simulink model "dynamic_simulation_control_old"  (R2017b)
settings: Solver=FixedStepAuto  StartTime=0.0  StopTime=20.0  FixedStep=1e-3  RelTol=1e-3
values from neighbouring files (symbols this model uses):
  B_env = [0;10;0]    [init_dynamic_sim.m]
  dth0 = [0; 0; 0]    [dynamic_simulation.m]    (also in init_dynamic_sim.m = dq0)
  fz0 = 0    [init_dynamic_sim.m]
  K = 0.015    [init_dynamic_sim.m]
  K_env = [0;100;0]    [init_dynamic_sim.m]
  Ki = 0.08    [init_dynamic_sim.m]
  Kj = [1;1;1]*5    [init_dynamic_sim.m]
  Kjd = [1;1;1]*0.1    [init_dynamic_sim.m]
  Kv = [2500;1500;2000]/256    [init_dynamic_sim.m]
  Kvi = [3000;900;1000]/65536    [init_dynamic_sim.m]
  Kx = [20;0;0]    [init_dynamic_sim.m]
  Kxi = [0;0;0]    [init_dynamic_sim.m]
  M_env = [0;1;0]    [init_dynamic_sim.m]
  ry0 = acos(r(1,1))    [init_dynamic_sim.m]
  th0 = 0    [DGM_youBot.m]    (also in DGM_youBot_sym.m; dynamic_simulation.m = q_dh - (q0_kuka - q_rob); init_dynamic_sim.m = theta_DH(2:4) - (q0 - KUKA_offset(2:4)))
  thmax = theta_DH - (qmin - KUKA_offset)    [init_dynamic_sim.m]
  thmin = theta_DH - (qmax - KUKA_offset)    [init_dynamic_sim.m]
  x0 = p0(1)    [init_dynamic_sim.m]    (also in jacobian_computation.m = 0.033)
  z0 = 0.3    [dynamic_simulation.m]    (also in init_dynamic_sim.m = p0(3); jacobian_computation.m = 0.147)
undefined symbols (not defined in the file or in its folder): p0
libraries: aerolibutil x1
settings Model: Creator=fortineau_vin  LastModifiedBy=fortineau_vin

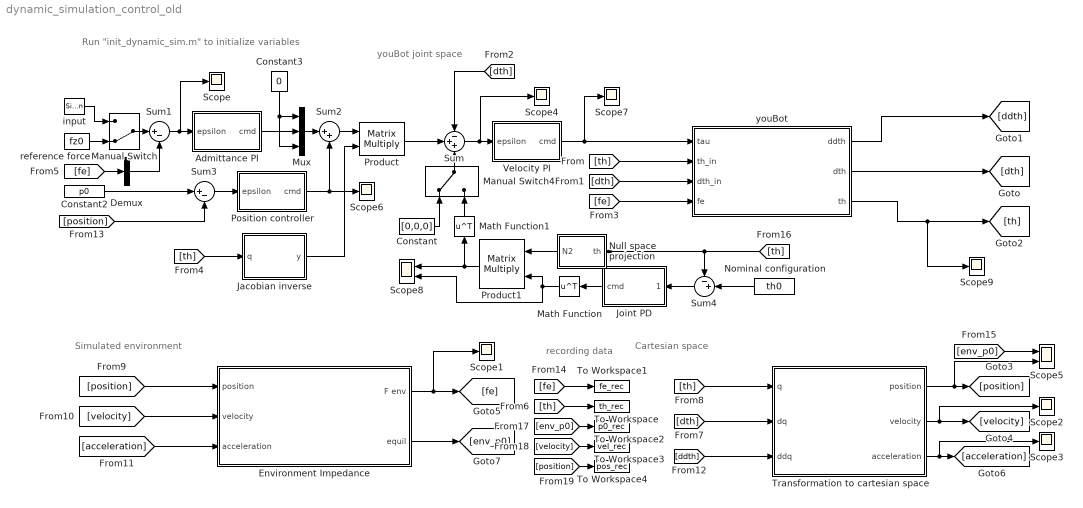
== system dynamic_simulation_control_old ==
  note: recording data
  note: Run "init_dynamic_sim.m" to initialize variables
  note: youBot joint space
  note: Simulated environment
  note: Cartesian space
  Admittance PI : Subsystem
  Constant : Constant  Value=[0,0,0]
  Constant2 : Constant  Value=p0
  Constant3 : Constant  Value=0
  Demux : Demux  Outputs=3
  "Environment Impedance " : Subsystem
  Jacobian inverse : MATLAB Function  TreatAsAtomicUnit=on
  Joint PD : Subsystem
  Manual Switch : ManualSwitch  CurrentSetting=0
  Manual Switch4 : ManualSwitch
  Math Function : Math  Operator=transpose  SaturateOnIntegerOverflow=on
  Math Function1 : Math  Operator=transpose  SaturateOnIntegerOverflow=on
  Mux : Mux  Inputs=3
  Nominal configuration : Constant  Value=th0
  Null space projection : Subsystem
  Position controller : Subsystem
  Product : Product  Multiplication=Matrix(*)
  Product1 : Product  Multiplication=Matrix(*)
  Scope{,1..4,6..7,9} (8 alike) : Scope
  Scope5 : Scope  NumInputPorts=2
  Scope8 : Scope  NumInputPorts=2
  Sum : Sum  Inputs=-++
  Sum1 : Sum  Inputs=|+-
  Sum2 : Sum  Inputs=|++
  Sum3 : Sum  Inputs=|+-
  Sum4 : Sum  Inputs=-+|
  To Workspace : ToWorkspace  VariableName=th_rec  SaveFormat=Structure  SampleTime=1e-3
      settings: Save2DSignal=2-D array (concatenate along first dimension)
  To Workspace1 : ToWorkspace  VariableName=fe_rec  SaveFormat=Structure  SampleTime=1e-3
      settings: Save2DSignal=2-D array (concatenate along first dimension)
  To Workspace2 : ToWorkspace  VariableName=p0_rec  SaveFormat=Structure  SampleTime=1e-3
      settings: Save2DSignal=2-D array (concatenate along first dimension)
  To Workspace3 : ToWorkspace  VariableName=vel_rec  SaveFormat=Structure  SampleTime=1e-3
      settings: Save2DSignal=2-D array (concatenate along first dimension)
  To Workspace4 : ToWorkspace  VariableName=pos_rec  SaveFormat=Structure  SampleTime=1e-3
      settings: Save2DSignal=2-D array (concatenate along first dimension)
  Transformation to cartesian space : Subsystem
  Velocity PI : Subsystem
  "input " : SignalGenerator  Amplitude=5  Frequency=0.9  Units=rad/sec
  reference force : Constant  Value=fz0
  youBot : Subsystem
  wires:
  Velocity PI/1(cmd) -> Scope7/1, youBot/1(tau)
  Sum/1 -> Scope4/1, Velocity PI/1(epsilon)
  [dth] -> Sum/1
  Jacobian inverse/1(y) -> Product/2
  Product/1 -> Sum/2
  Sum1/1 -> Admittance PI/1(epsilon), Scope/1
  [th] -> Jacobian inverse/1(q)
  [position] -> "Environment Impedance "/1(position)
  [velocity] -> "Environment Impedance "/2(velocity)
  [acceleration] -> "Environment Impedance "/3(acceleration)
  [dth] -> Transformation to cartesian space/2(dq)
  [th] -> Transformation to cartesian space/1(q)
  [ddth] -> Transformation to cartesian space/3(ddq)
  Transformation to cartesian space/1(position) -> Scope5/2, [position]
  Sum2/1 -> Product/1
  Position controller/1(cmd) -> Scope6/1, Sum2/2
  Sum3/1 -> Position controller/1(epsilon)
  Constant2/1 -> Sum3/1
  [position] -> Sum3/2
  [fe] -> Demux/1
  Admittance PI/1(cmd) -> Mux/2
  Mux/1 -> Sum2/1
  Constant3/1 -> Mux/3, Mux/1
  [th] -> To Workspace/1
  Manual Switch/1 -> Sum1/1
  reference force/1 -> Manual Switch/2
  "input "/1 -> Manual Switch/1
  [fe] -> To Workspace1/1
  Demux/2 -> Sum1/2
  [th] -> youBot/2(th_in)
  [dth] -> youBot/3(dth_in)
  [fe] -> youBot/4(fe)
  youBot/1(ddth) -> [ddth]
  youBot/2(dth) -> [dth]
  youBot/3(th) -> Scope9/1, [th]
  Transformation to cartesian space/2(velocity) -> [velocity], Scope2/1
  Transformation to cartesian space/3(acceleration) -> [acceleration], Scope3/1
  "Environment Impedance "/2(equil) -> [env_p0]
  [env_p0] -> Scope5/1
  Sum4/1 -> Joint PD/1(epsilon)
  Nominal configuration/1 -> Sum4/2
  Product1/1 -> Scope8/1, Math Function1/1
  Null space projection/1(N2) -> Product1/1
  [th] -> Null space projection/1(th), Sum4/1
  Joint PD/1(cmd) -> Math Function/1
  Math Function/1 -> Scope8/2, Product1/2
  Manual Switch4/1 -> Sum/3
  Math Function1/1 -> Manual Switch4/2
  Constant/1 -> Manual Switch4/1
  "Environment Impedance "/1(F env) -> [fe], Scope1/1
  [env_p0] -> To Workspace2/1
  [velocity] -> To Workspace3/1
  [position] -> To Workspace4/1

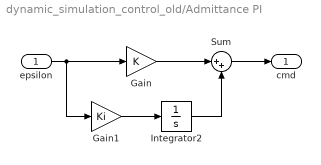
== system dynamic_simulation_control_old/Admittance PI ==
  epsilon : Inport
  Gain : Gain  Gain=K
  Gain1 : Gain  Gain=Ki
  Integrator2 : Integrator
  Sum : Sum  Inputs=|++
  cmd : Outport
  wires:
  Integrator2/1 -> Sum/2
  Gain/1 -> Sum/1
  Gain1/1 -> Integrator2/1
  epsilon/1 -> Gain/1, Gain1/1
  Sum/1 -> cmd/1

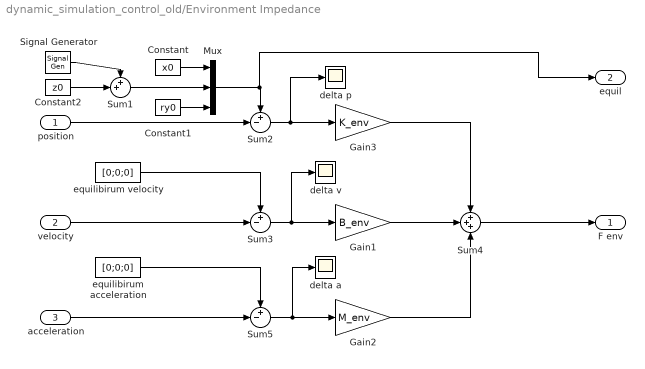
== system dynamic_simulation_control_old/Environment Impedance  ==
  position : Inport
  velocity : Inport  Port=2
  acceleration : Inport  Port=3
  Constant : Constant  Value=x0
  Constant1 : Constant  Value=ry0
  Constant2 : Constant  Value=z0
  Gain1 : Gain  Gain=B_env
  Gain2 : Gain  Gain=M_env
  Gain3 : Gain  Gain=K_env
  Mux : Mux  Inputs=3
  Signal Generator : SignalGenerator  Amplitude=0.01  Frequency=0.9
  Sum1 : Sum  Inputs=++|
  Sum2 : Sum  Inputs=+-|
  Sum3 : Sum  Inputs=+-|
  Sum4 : Sum  Inputs=+++
  Sum5 : Sum  Inputs=+-|
  delta a : Scope
  delta p : Scope
  delta v : Scope
  equilibirum acceleration : Constant  Value=[0;0;0]
  equilibirum velocity : Constant  Value=[0;0;0]
  F env : Outport
  equil : Outport  Port=2
  wires:
  Gain3/1 -> Sum4/1
  velocity/1 -> Sum3/2
  position/1 -> Sum2/2
  Gain2/1 -> Sum4/3
  equilibirum velocity/1 -> Sum3/1
  Sum3/1 -> delta v/1, Gain1/1
  Sum4/1 -> F env/1
  acceleration/1 -> Sum5/2
  Sum5/1 -> delta a/1, Gain2/1
  Gain1/1 -> Sum4/2
  equilibirum acceleration/1 -> Sum5/1
  Sum2/1 -> delta p/1, Gain3/1
  Constant/1 -> Mux/1
  Constant1/1 -> Mux/3
  Mux/1 -> equil/1, Sum2/1
  Sum1/1 -> Mux/2
  Constant2/1 -> Sum1/2
  Signal Generator/1 -> Sum1/1

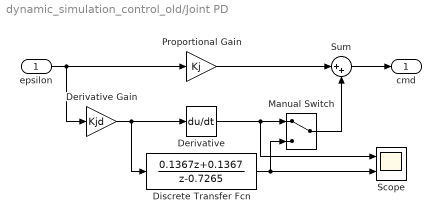
== system dynamic_simulation_control_old/Joint PD ==
  epsilon : Inport
  " Derivative Gain" : Gain  Gain=Kjd
  Derivative : Derivative
  Discrete Transfer Fcn : DiscreteTransferFcn  Numerator=[0.1367 0.1367]  Denominator=[1 -0.7265]
  Manual Switch : ManualSwitch
  Proportional Gain : Gain  Gain=Kj
  Scope : Scope  NumInputPorts=2
  Sum : Sum  Inputs=|++
  cmd : Outport
  wires:
  Sum/1 -> cmd/1
  epsilon/1 -> " Derivative Gain"/1, Proportional Gain/1
  " Derivative Gain"/1 -> Derivative/1, Discrete Transfer Fcn/1
  Proportional Gain/1 -> Sum/1
  Derivative/1 -> Scope/1, Manual Switch/1
  Manual Switch/1 -> Sum/2
  Discrete Transfer Fcn/1 -> Scope/2, Manual Switch/2

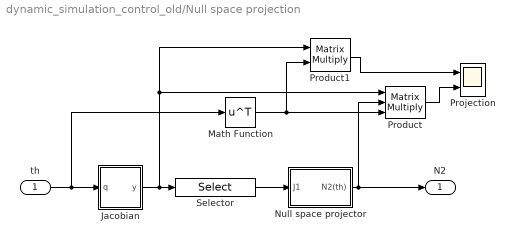
== system dynamic_simulation_control_old/Null space projection ==
  th : Inport
  Jacobian : MATLAB Function  TreatAsAtomicUnit=on
  Math Function : Math  Operator=transpose  SaturateOnIntegerOverflow=on
  Null space projector : Subsystem
  Product : Product  Inputs=3  Multiplication=Matrix(*)
  Product1 : Product  Multiplication=Matrix(*)
  Projection : Scope  NumInputPorts=2
  Selector : Selector  NumberOfDimensions=2  InputPortWidth=3  IndexOptions=Index vector (dialog),Index vector (dialog)  Indices=2,[1 2 3]  OutputSizes=1,1
  N2 : Outport
  wires:
  Null space projector/1(N2(th)) -> N2/1, Product/2
  th/1 -> Math Function/1, Jacobian/1(q)
  Jacobian/1(y) -> Product1/1, Product/1, Selector/1
  Selector/1 -> Null space projector/1(J1)
  Math Function/1 -> Product1/2, Product/3
  Product/1 -> Projection/2
  Product1/1 -> Projection/1

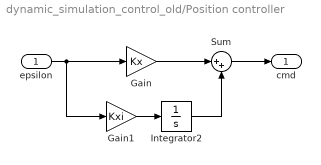
== system dynamic_simulation_control_old/Position controller ==
  epsilon : Inport
  Gain : Gain  Gain=Kx
  Gain1 : Gain  Gain=Kxi
  Integrator2 : Integrator
  Sum : Sum  Inputs=|++
  cmd : Outport
  wires:
  Sum/1 -> cmd/1
  epsilon/1 -> Gain1/1, Gain/1
  Gain1/1 -> Integrator2/1
  Gain/1 -> Sum/1
  Integrator2/1 -> Sum/2

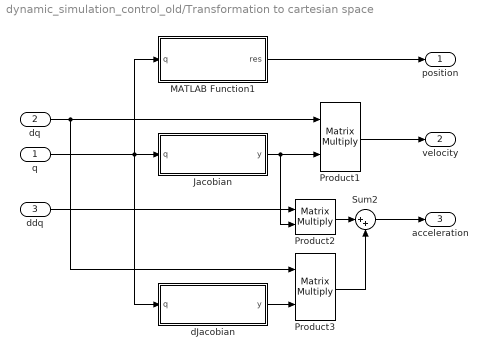
== system dynamic_simulation_control_old/Transformation to cartesian space ==
  q : Inport
  dq : Inport  Port=2
  ddq : Inport  Port=3
  Jacobian : MATLAB Function  TreatAsAtomicUnit=on
  MATLAB Function1 : MATLAB Function  TreatAsAtomicUnit=on
  Product1 : Product  Multiplication=Matrix(*)
  Product2 : Product  Multiplication=Matrix(*)
  Product3 : Product  Multiplication=Matrix(*)
  Sum2 : Sum  Inputs=|++
  dJacobian : MATLAB Function  TreatAsAtomicUnit=on
  position : Outport
  velocity : Outport  Port=2
  acceleration : Outport  Port=3
  wires:
  MATLAB Function1/1(res) -> position/1
  q/1 -> dJacobian/1(q), MATLAB Function1/1(q), Jacobian/1(q)
  Product1/1 -> velocity/1
  Product2/1 -> Sum2/1
  dJacobian/1(y) -> Product3/2
  Sum2/1 -> acceleration/1
  ddq/1 -> Product2/1
  Product3/1 -> Sum2/2
  dq/1 -> Product1/1, Product3/1
  Jacobian/1(y) -> Product2/2, Product1/2

== system dynamic_simulation_control_old/Velocity PI ==
  epsilon : Inport
  Gain : Gain  Gain=Kv
  Gain1 : Gain  Gain=Kvi
  Integrator2 : Integrator
  Sum : Sum  Inputs=|++
  cmd : Outport
  wires:
  Sum/1 -> cmd/1
  epsilon/1 -> Gain1/1, Gain/1
  Gain1/1 -> Integrator2/1
  Gain/1 -> Sum/1
  Integrator2/1 -> Sum/2

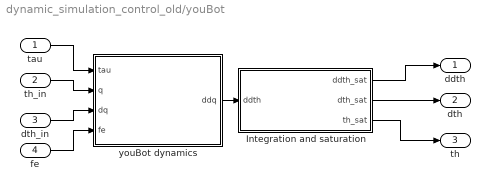
== system dynamic_simulation_control_old/youBot ==
  tau : Inport
  th_in : Inport  Port=2
  dth_in : Inport  Port=3
  fe : Inport  Port=4
  Integration and saturation : Subsystem
  youBot dynamics : Subsystem
  ddth : Outport
  dth : Outport  Port=2
  th : Outport  Port=3
  wires:
  tau/1 -> youBot dynamics/1(tau)
  youBot dynamics/1(ddq) -> Integration and saturation/1(ddth)
  dth_in/1 -> youBot dynamics/3("dq ")
  th_in/1 -> youBot dynamics/2("q ")
  fe/1 -> youBot dynamics/4(fe)
  Integration and saturation/3(th_sat) -> th/1
  Integration and saturation/1(ddth_sat) -> ddth/1
  Integration and saturation/2(dth_sat) -> dth/1

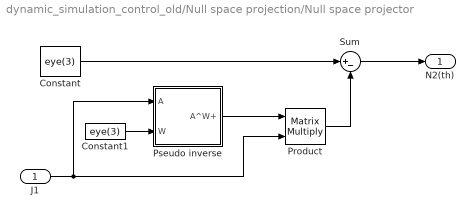
== system dynamic_simulation_control_old/Null space projection/Null space projector ==
  J1 : Inport
  Constant : Constant  Value=eye(3)  VectorParams1D=off
  Constant1 : Constant  Value=eye(3)  VectorParams1D=off
  Product : Product  Multiplication=Matrix(*)
  Pseudo inverse : Subsystem
  Sum : Sum  Inputs=|+-
  N2(th) : Outport
  wires:
  Constant/1 -> Sum/1
  Constant1/1 -> Pseudo inverse/2(W)
  J1/1 -> Pseudo inverse/1(A), Product/2
  Pseudo inverse/1(A^W+) -> Product/1
  Product/1 -> Sum/2
  Sum/1 -> N2(th)/1

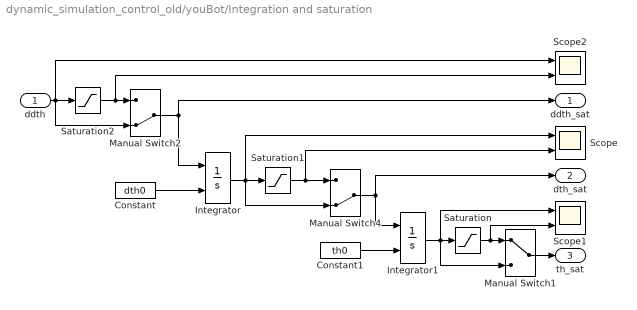
== system dynamic_simulation_control_old/youBot/Integration and saturation ==
  ddth : Inport
  Constant : Constant  Value=dth0
  Constant1 : Constant  Value=th0
  Integrator : Integrator  InitialConditionSource=external
  Integrator1 : Integrator  InitialConditionSource=external
  Manual Switch1 : ManualSwitch
  Manual Switch2 : ManualSwitch  CurrentSetting=0
  Manual Switch4 : ManualSwitch  CurrentSetting=0
  Saturation : Saturate  UpperLimit=thmax(2:4)'  LowerLimit=thmin(2:4)'
  Saturation1 : Saturate
  Saturation2 : Saturate
  Scope : Scope  NumInputPorts=2
  Scope1 : Scope  NumInputPorts=2
  Scope2 : Scope  NumInputPorts=2
  ddth_sat : Outport
  dth_sat : Outport  Port=2
  th_sat : Outport  Port=3
  wires:
  Manual Switch2/1 -> ddth_sat/1, Integrator/1
  Manual Switch1/1 -> th_sat/1
  Manual Switch4/1 -> Integrator1/1, dth_sat/1
  ddth/1 -> Scope2/1, Manual Switch2/2, Saturation2/1
  Saturation2/1 -> Scope2/2, Manual Switch2/1
  Saturation1/1 -> Scope/2, Manual Switch4/1
  Saturation/1 -> Scope1/2, Manual Switch1/1
  Constant/1 -> Integrator/2
  Integrator/1 -> Scope/1, Manual Switch4/2, Saturation1/1
  Integrator1/1 -> Scope1/1, Manual Switch1/2, Saturation/1
  Constant1/1 -> Integrator1/2

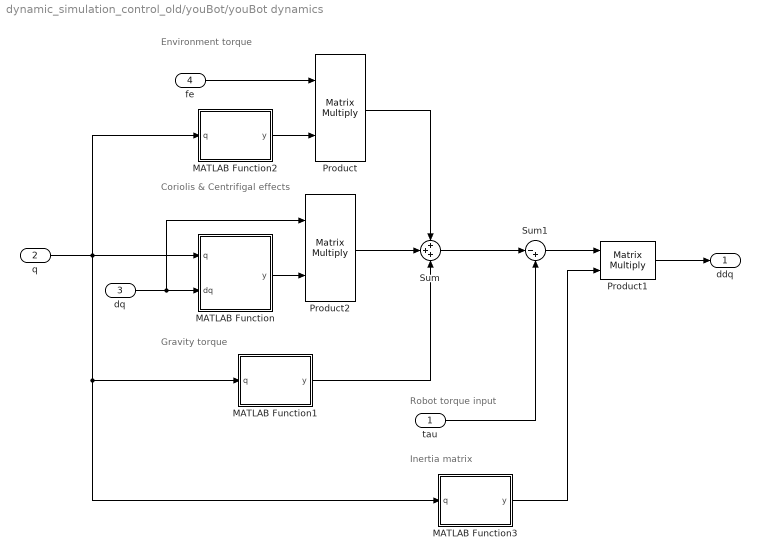
== system dynamic_simulation_control_old/youBot/youBot dynamics ==
  note: Coriolis & Centrifigal effects
  note: Gravity torque
  note: Environment torque
  note: Robot torque input
  note: Inertia matrix
  tau : Inport
  "q " : Inport  Port=2
  "dq " : Inport  Port=3
  fe : Inport  Port=4
  MATLAB Function : MATLAB Function  TreatAsAtomicUnit=on
  MATLAB Function1 : MATLAB Function  TreatAsAtomicUnit=on
  MATLAB Function2 : MATLAB Function  TreatAsAtomicUnit=on
  MATLAB Function3 : MATLAB Function  TreatAsAtomicUnit=on
  Product : Product  Multiplication=Matrix(*)
  Product1 : Product  Multiplication=Matrix(*)
  Product2 : Product  Multiplication=Matrix(*)
  Sum : Sum  Inputs=+++
  Sum1 : Sum  Inputs=|-+
  ddq : Outport
  wires:
  MATLAB Function2/1(y) -> Product/2
  "dq "/1 -> Product2/1, MATLAB Function/2(dq)
  "q "/1 -> MATLAB Function3/1(q), MATLAB Function1/1(q), MATLAB Function/1(q), MATLAB Function2/1(q)
  fe/1 -> Product/1
  Product/1 -> Sum/1
  Product1/1 -> ddq/1
  MATLAB Function1/1(y) -> Sum/3
  Sum/1 -> Sum1/1
  tau/1 -> Sum1/2
  Product2/1 -> Sum/2
  Sum1/1 -> Product1/1
  MATLAB Function3/1(y) -> Product1/2
  MATLAB Function/1(y) -> Product2/2

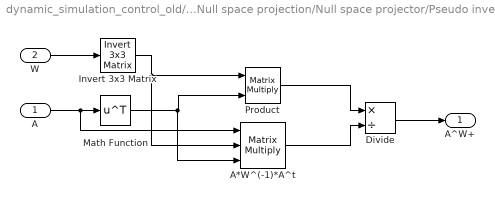
== system dynamic_simulation_control_old/Null space projection/Null space projector/Pseudo inverse ==
  A : Inport
  W : Inport  Port=2
  A*W^(-1)*A^t : Product  Inputs=3  Multiplication=Matrix(*)
  Divide : Product  Inputs=*/
  Invert 3x3 Matrix : aerolibutil/Invert  3x3 Matrix
  Math Function : Math  Operator=transpose  SaturateOnIntegerOverflow=on
  Product : Product  Multiplication=Matrix(*)
  A^W+ : Outport
  wires:
  W/1 -> Invert 3x3 Matrix/1
  A/1 -> A*W^(-1)*A^t/1, Math Function/1
  Math Function/1 -> A*W^(-1)*A^t/3, Product/2
  Invert 3x3 Matrix/1 -> A*W^(-1)*A^t/2, Product/1
  Product/1 -> Divide/1
  A*W^(-1)*A^t/1 -> Divide/2
  Divide/1 -> A^W+/1

== matlab function dynamic_simulation_control_old/youBot/youBot dynamics/MATLAB Function1 ==
  data: q input; y output
function y = G_sim(q)
q1 = q(1);
q2 = q(2);
q3 = q(3);
y = G_3DOF(q1,q2,q3);

== matlab function dynamic_simulation_control_old/youBot/youBot dynamics/MATLAB Function ==
  data: q input; y output; dq input
function y = C_sim(q,dq)
q2 = q(2);
q3 = q(3);
dq1 = dq(1);
dq2 = dq(2);
dq3 = dq(3);
y = C_3DOF(dq1,dq2,dq3,q2,q3);

== matlab function dynamic_simulation_control_old/youBot/youBot dynamics/MATLAB Function2 ==
  data: q input; y output
function y = tJ_sim(q)
q1 = q(1);
q2 = q(2);
q3 = q(3);
y = J0E_3DOF(q1,q2,q3)';

== matlab function dynamic_simulation_control_old/youBot/youBot dynamics/MATLAB Function3 ==
  data: q input; y output
function y = iM_sim(q)
q2 = q(2);
q3 = q(3);
y = iM_3DOF(q2,q3);

== matlab function dynamic_simulation_control_old/Jacobian inverse ==
  data: q input; y output
function y = iJ(q)
q1 = q(1);
q2 = q(2);
q3 = q(3);
y = iJ0E_3DOF(q1,q2,q3);

== matlab function dynamic_simulation_control_old/Transformation to cartesian space/dJacobian ==
  data: q input; y output
function y = dJ(q)
q1 = q(1);
q2 = q(2);
q3 = q(3);
y = dJ0E_3DOF(q1,q2,q3);

== matlab function dynamic_simulation_control_old/Transformation to cartesian space/Jacobian ==
  data: q input; y output
function y = J(q)
q1 = q(1);
q2 = q(2);
q3 = q(3);
y = J0E_3DOF(q1,q2,q3);

== matlab function dynamic_simulation_control_old/Transformation to cartesian space/MATLAB Function1 ==
  data: q input; res output
function res = forwardKinematics(q)

x0 = 0;
le = 0.1;

[p,r,~] = DGM_youBot(q, x0, le);

x  = p(1);
z  = p(3);
ry = acos(r(1,1));

res = [x,z,ry]';

== matlab function dynamic_simulation_control_old/Null space projection/Jacobian ==
  data: q input; y output
function y = J(q)
q1 = q(1);
q2 = q(2);
q3 = q(3);
y = J0E_3DOF(q1,q2,q3);
